simulink model "sim2ndorderdsm"  (R2021b)
settings: Solver=VariableStepAuto  StartTime=0.0  StopTime=10  RelTol=1e-3
settings Model: Creator=chand  LastModifiedBy=chand
settings DataIOCC: ExternalInput=u  ReturnWorkspaceOutputs=off
settings DebuggingCC: AlgebraicLoopMsg=none

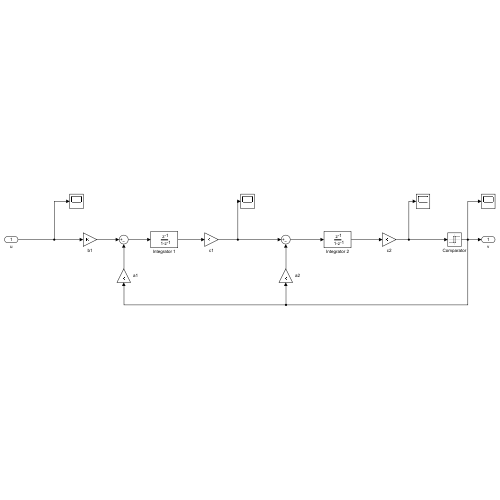
[thumbnail: Simulink's stored preview of the top-level diagram]
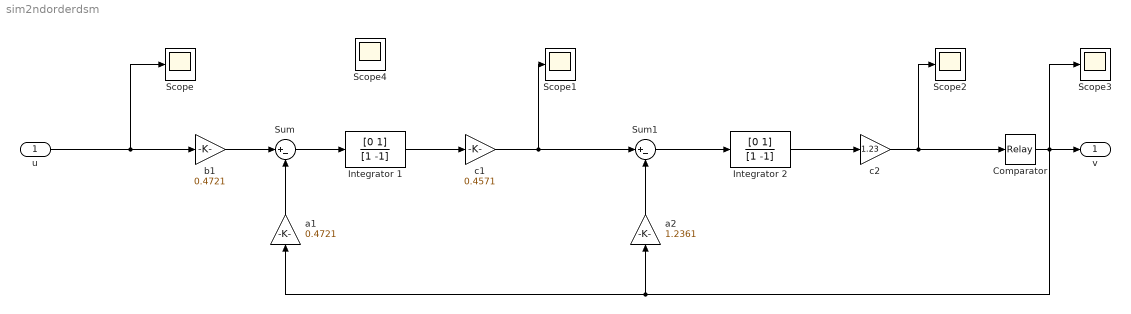
== system sim2ndorderdsm ==
  u : Inport
  Comparator : Relay  OffOutputValue=-1
  Integrator 1 : DiscreteFilter  Numerator=[0 1]  Denominator=[1 -1]
  Integrator 2 : DiscreteFilter  Numerator=[0 1]  Denominator=[1 -1]
  Scope{,1..4} (5 alike) : Scope
  Sum : Sum  Inputs=|+-
  Sum1 : Sum  Inputs=|+-
  a1 : Gain  Gain=0.4721
  a2 : Gain  Gain=1.2361
  b1 : Gain  Gain=0.4721
  c1 : Gain  Gain=0.4571
  c2 : Gain  Gain=1.23
  v : Outport
  wires:
  b1/1 -> Sum/1
  a1/1 -> Sum/2
  a2/1 -> Sum1/2
  Sum1/1 -> Integrator 2/1
  c1/1 -> Scope1/1, Sum1/1
  Integrator 1/1 -> c1/1
  Sum/1 -> Integrator 1/1
  Integrator 2/1 -> c2/1
  c2/1 -> Scope2/1, Comparator/1
  Comparator/1 -> Scope3/1, a1/1, a2/1, v/1
  u/1 -> Scope/1, b1/1
